simulink model "gForce_data_acquisition_ccOnline_ROS_v2_1_R2020a"  (R2022a)
settings: Solver=FixedStepAuto  StartTime=0.0  StopTime=inf  FixedStep=0.001  RelTol=1e-3
values from neighbouring files (symbols this model uses):
  k_ext = sum(u_ext)/diff_range_2    [fnc_to_be_implemented.m]
  k_flex = sum(u_flex)/diff_range_2    [fnc_to_be_implemented.m]
  M_pinv = pinv(M)    [fnc_to_be_implemented.m]
undefined symbols (not defined in the file or in its folder): gForceBLE, magnitude, W, X, Y, Z
libraries: dspfdesign x16, dspstat3 x8, robotlib x4
settings Model: SimulationMode=accelerator  Creator=Armando  LastModifiedBy=Armando
settings SolverCC: AlgebraicLoopSolver=TrustRegion
settings OptimizationCC: EnhancedBackFolding=on  PassReuseOutputArgsThreshold=0  MaxStackSize=64  OptimizeBlockOrder=speed  DifferentSizesBufferReuse=on  OptimizationCustomize=off
settings DebuggingCC: ParameterTunabilityLossMsg=error  UnconnectedInputMsg=warning  UnconnectedOutputMsg=warning  UnconnectedLineMsg=warning  SFMachineParentedDataDiag=warning
settings HardwareCC: ProdBitPerPointer=32  ProdBitPerSizeT=32  ProdBitPerPtrDiffT=32  ProdLargestAtomicFloat=None  ProdIntDivRoundTo=Undefined  ProdEndianess=Unspecified  ProdWordSize=32  ProdHWDeviceType=Generic->Unspecified (assume 32-bit Generic)  UseEmbeddedCoderFeatures=off
settings SFSimCC: MATLABDynamicMemAlloc=off  SimTargetLang=C++
settings RTWCC: SystemTargetFile=ert.tlc  HardwareBoard=Robot Operating System (ROS)  TLCOptions="-aInlineSetEventsForThisBaseRateFcn=TLC_FALSE -aSuppressMultiTaskScheduler=TLC_FALSE  -aRateBasedStepFcn=0"  TemplateMakefile=ert_default_tmf  Toolchain=Catkin  TargetLang=C++
settings CodeAppCC: ForceParamTrailComments=on  OperatorAnnotations=on
settings ERTTargetCC: ERTCustomFileBanners=off  SupportContinuousTime=on  SupportNonInlinedSFcns=on  RemoveResetFunc=off  ModelStepFunctionPrototypeControlCompliant=off

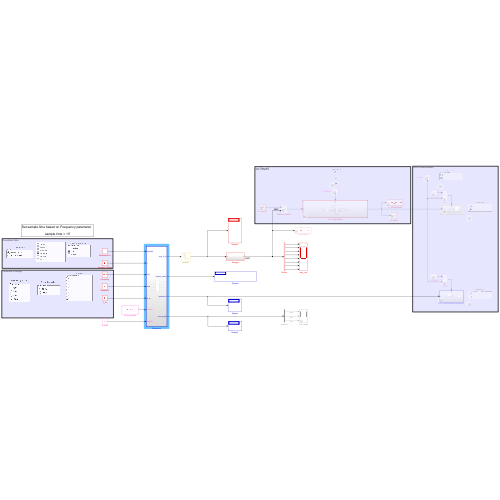
[thumbnail: Simulink's stored preview of the top-level diagram]
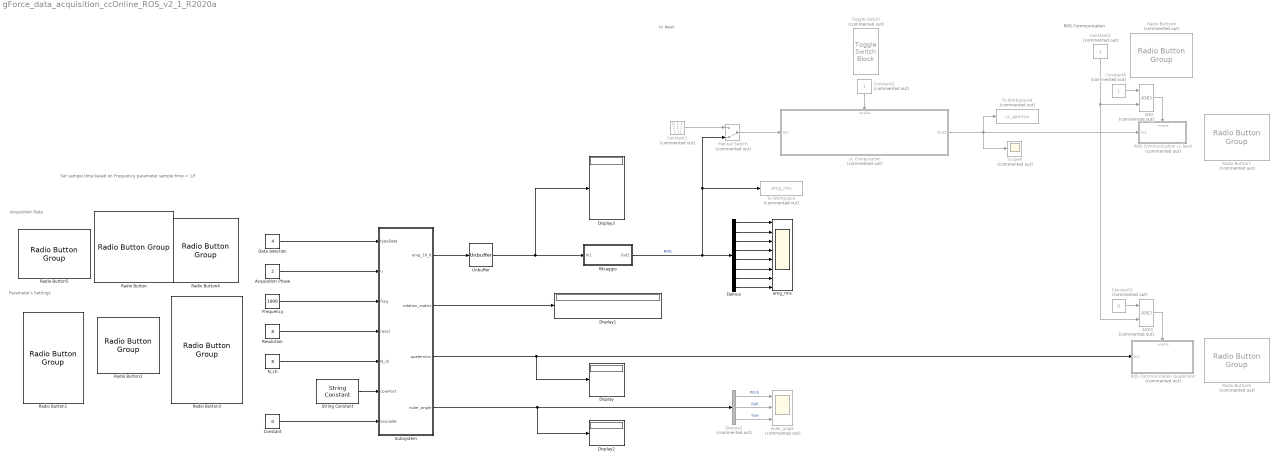
== system gForce_data_acquisition_ccOnline_ROS_v2_1_R2020a ==
  note: cc level
  note: Acquisition Data
  note: Parameter's Settings
  note: Set sample time based on Frequency parameter
      |
      | sample time = 1/f
  note: ROS Communication
  AND : Logic  Commented=on  IconShape=distinctive  AllPortsSameDT=off  OutDataTypeStr=boolean
  AND1 : Logic  Commented=on  IconShape=distinctive  AllPortsSameDT=off  OutDataTypeStr=boolean
  Acquisition Phase : Constant  Value=2  SampleTime=0.001
  Constant : Constant  Value=0
  Constant1 : Constant  Commented=on  Value=[1 1 1 1 1 1 1 1]  SampleTime=0.001
  Constant2 : Constant  Commented=on
  Constant3 : Constant  Commented=on
  Constant4 : Constant  Commented=on
  Constant5 : Constant  Commented=on  Value=0
  Data selection : Constant  Value=4  SampleTime=0.001
  Demux : Demux  Outputs=8
  Demux2 : Demux  Commented=on  Outputs=3
  Display{,1..3} (4 alike) : Display
  Frequency : Constant  Value=1000  SampleTime=0.001
  Manual Switch : ManualSwitch  Commented=on  CurrentSetting=0
  N_ch : Constant  Value=8  SampleTime=0.001
  ROS Communication cc level : Subsystem  Commented=on  TreatAsAtomicUnit=on
  ROS Communication quaternion : Subsystem  Commented=on
  Radio Button : RadioButtonGroup  SelectedLabel=EMG Raw Data  ButtonGroupName=Data Selection
      settings: Values={{'Euler Angle', 'Quaternion', 'Rotation Matrix', 'EMG Raw Data', 'EMG + Euler', 'EMG + Quat'}, [1 2 3 4 5 6]}
  Radio Button1 : RadioButtonGroup  SelectedLabel=1000  ButtonGroupName=Frequency
      settings: Values={{'100', '500', '650', '1000'}, [100 500 650 1000]}
  Radio Button2 : RadioButtonGroup  SelectedLabel=8 byte  ButtonGroupName=Resolution
      settings: Values={{'8 byte', '12 byte'}, [8 12]}
  Radio Button3 : RadioButtonGroup  SelectedLabel=8  ButtonGroupName=Numer of channels to read
      settings: Values={{'1', '2', '3', '4', '5', '6', '7', '8'}, [1 2 3 4 5 6 7 8]}
  Radio Button4 : RadioButtonGroup  SelectedLabel=Stop  ButtonGroupName=Acquisition Phase
      settings: Values={{'Acquisition', 'Stop', 'cc-level'}, [1 2 3]}
  Radio Button5 : RadioButtonGroup  SelectedLabel=gForceBLE(5CB7)  ButtonGroupName=Bracialet
      settings: Values={{'gForceBLE(5CB7)', 'gForcePro+(3BB9)'}, [0 1]}
  Radio Button6 : RadioButtonGroup  Commented=on  SelectedLabel=ON  ButtonGroupName=ROS Communication
      settings: Values={{'OFF', 'ON'}, [0 1]}
  Radio Button7 : RadioButtonGroup  Commented=on  SelectedLabel=ON  ButtonGroupName=ROS Communication cc value
      settings: Values={{'OFF', 'ON'}, [0 1]}
  Radio Button8 : RadioButtonGroup  Commented=on  SelectedLabel=OFF  ButtonGroupName=ROS Communication quaternion
      settings: Values={{'OFF', 'ON'}, [0 1]}
  Resolution : Constant  Value=8  SampleTime=0.001
  Scope6 : Scope  Commented=on
  String Constant : StringConstant  String="\"COM3\""
  Subsystem : Subsystem  TreatAsAtomicUnit=on  SystemSampleTime=0.016
  To Workspace : ToWorkspace  Commented=on  VariableName=emg_rms  SaveFormat=Timeseries  SampleTime=-1
  To Workspace4 : ToWorkspace  Commented=on  VariableName=cc_gamma  SaveFormat=Timeseries  SampleTime=-1
  Toggle Switch : ToggleSwitchBlock  Commented=on
      settings: Values={{'Off', 'On'}, [0 1]}
  Unbuffer : Unbuffer
  cc Computation : Subsystem  Commented=on
  emg_rms : Scope  NumInputPorts=8
  euler_angle : Scope  Commented=on  NumInputPorts=3
  filtraggio : Subsystem
  wires:
  Demux/8 -> emg_rms/8
  Demux2/1 -> euler_angle/1  "Pitch"
  Demux2/2 -> euler_angle/2  "Roll"
  Demux2/3 -> euler_angle/3  "Yaw"
  Subsystem/1(emg_16_8) -> Unbuffer/1
  Data selection/1 -> Subsystem/1(typeData)
  Acquisition Phase/1 -> Subsystem/2(u)
  Frequency/1 -> Subsystem/3(freq)
  Resolution/1 -> Subsystem/4(resol)
  N_ch/1 -> Subsystem/5(N_ch)
  Unbuffer/1 -> Display3/1, filtraggio/1(In1)
  Demux/1 -> emg_rms/1
  Demux/2 -> emg_rms/2
  Demux/3 -> emg_rms/3
  Demux/4 -> emg_rms/4
  Demux/5 -> emg_rms/5
  Demux/6 -> emg_rms/6
  Demux/7 -> emg_rms/7
  Subsystem/2(rotation_matrix) -> Display1/1
  String Constant/1 -> Subsystem/6(comPort)
  Constant/1 -> Subsystem/7(bracialet)
  Constant1/1 -> Manual Switch/1
  filtraggio/1(Out1) -> Manual Switch/2, To Workspace/1, Demux/1  "RMS"
  Manual Switch/1 -> cc Computation/1(In1)
  Constant2/1 -> cc Computation/Enable
  cc Computation/1(Out1) -> Scope6/1, ROS Communication cc level/1(In1), To Workspace4/1
  Subsystem/3(quaternion) -> ROS Communication quaternion/1(In1), Display/1
  AND/1 -> ROS Communication cc level/Enable
  AND1/1 -> ROS Communication quaternion/Enable
  Constant4/1 -> AND/1
  Constant5/1 -> AND1/1
  Constant3/1 -> AND1/2, AND/2
  Subsystem/4(euler_angle) -> Display2/1, Demux2/1

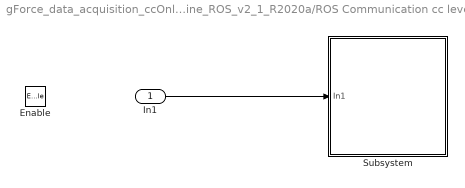
== system gForce_data_acquisition_ccOnline_ROS_v2_1_R2020a/ROS Communication cc level ==
  In1 : Inport
  Enable : EnablePort
  Subsystem : Subsystem  TreatAsAtomicUnit=on  SystemSampleTime=0.01
  wires:
  In1/1 -> Subsystem/1(In1)

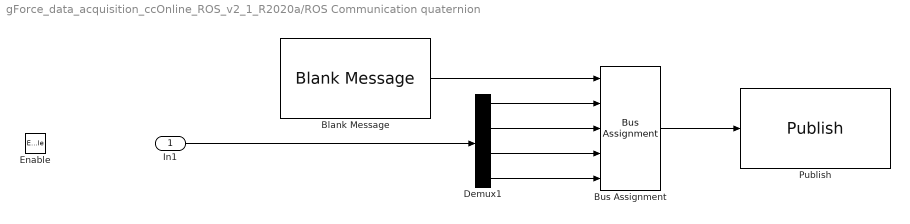
== system gForce_data_acquisition_ccOnline_ROS_v2_1_R2020a/ROS Communication quaternion ==
  In1 : Inport
  Enable : EnablePort
  Blank Message : robotlib/Blank Message  messageClass=Message  entityType=geometry_msgs/Quaternion  messageType=geometry_msgs/Quaternion  SampleTime=inf  legacyBusStruct=off
  Bus Assignment : BusAssignment  AssignedSignals=W,X,Y,Z
  Demux1 : Demux
  Publish : robotlib/Publish  topicSource=Specify your own  topic=/gForce_quaternion  messageType=geometry_msgs/Quaternion  legacyBusStruct=off  messageQueueLength=1
  wires:
  Bus Assignment/1 -> Publish/1
  Blank Message/1 -> Bus Assignment/1
  Demux1/4 -> Bus Assignment/5
  Demux1/1 -> Bus Assignment/2
  Demux1/2 -> Bus Assignment/3
  Demux1/3 -> Bus Assignment/4
  In1/1 -> Demux1/1

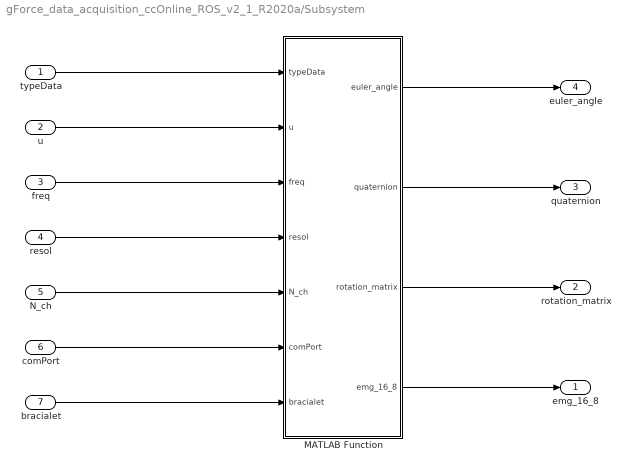
== system gForce_data_acquisition_ccOnline_ROS_v2_1_R2020a/Subsystem ==
  typeData : Inport
  u : Inport  Port=2
  freq : Inport  Port=3
  resol : Inport  Port=4
  N_ch : Inport  Port=5
  comPort : Inport  Port=6
  bracialet : Inport  Port=7
  MATLAB Function : MATLAB Function  TreatAsAtomicUnit=on  SystemSampleTime=0.016
  emg_16_8 : Outport
  rotation_matrix : Outport  Port=2
  quaternion : Outport  Port=3
  euler_angle : Outport  Port=4
  wires:
  N_ch/1 -> MATLAB Function/5(N_ch)
  freq/1 -> MATLAB Function/3(freq)
  resol/1 -> MATLAB Function/4(resol)
  u/1 -> MATLAB Function/2(u)
  MATLAB Function/4(emg_16_8) -> emg_16_8/1
  typeData/1 -> MATLAB Function/1(typeData)
  MATLAB Function/3(rotation_matrix) -> rotation_matrix/1
  MATLAB Function/2(quaternion) -> quaternion/1
  MATLAB Function/1(euler_angle) -> euler_angle/1
  comPort/1 -> MATLAB Function/6(comPort)
  bracialet/1 -> MATLAB Function/7(bracialet)

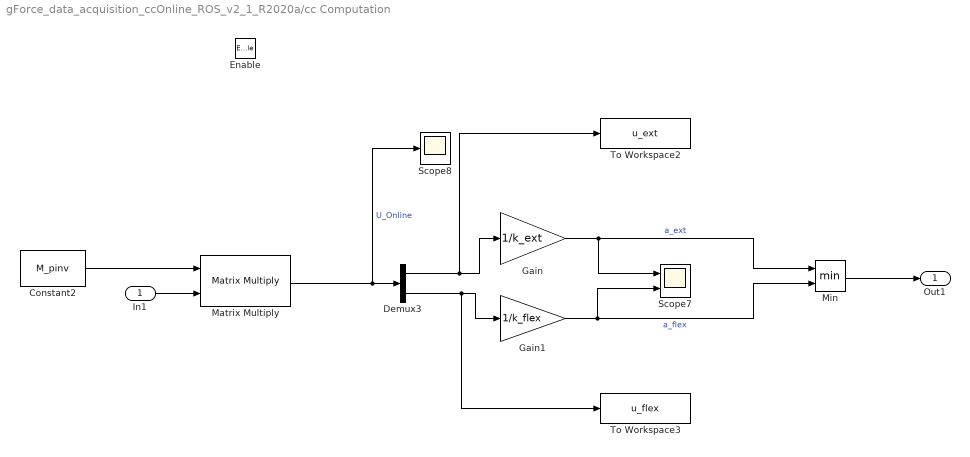
== system gForce_data_acquisition_ccOnline_ROS_v2_1_R2020a/cc Computation ==
  In1 : Inport
  Enable : EnablePort
  Constant2 : Constant  Value=M_pinv  SampleTime=0.001
  Demux3 : Demux  Outputs=2
  Gain : Gain  Gain=1/k_ext
  Gain1 : Gain  Gain=1/k_flex
  Matrix Multiply : Product  Multiplication=Matrix(*)
  Min : MinMax  Inputs=2
  Scope7 : Scope  NumInputPorts=2
  Scope8 : Scope
  To Workspace2 : ToWorkspace  VariableName=u_ext  SaveFormat=Timeseries  SampleTime=-1
  To Workspace3 : ToWorkspace  VariableName=u_flex  SaveFormat=Timeseries  SampleTime=-1
  Out1 : Outport
  wires:
  Gain1/1 -> Scope7/2, Min/2  "a_flex"
  Matrix Multiply/1 -> Demux3/1, Scope8/1  "U_Online"
  Constant2/1 -> Matrix Multiply/1
  Gain/1 -> Scope7/1, Min/1  "a_ext"
  Demux3/1 -> To Workspace2/1, Gain/1
  Min/1 -> Out1/1
  Demux3/2 -> To Workspace3/1, Gain1/1
  In1/1 -> Matrix Multiply/2

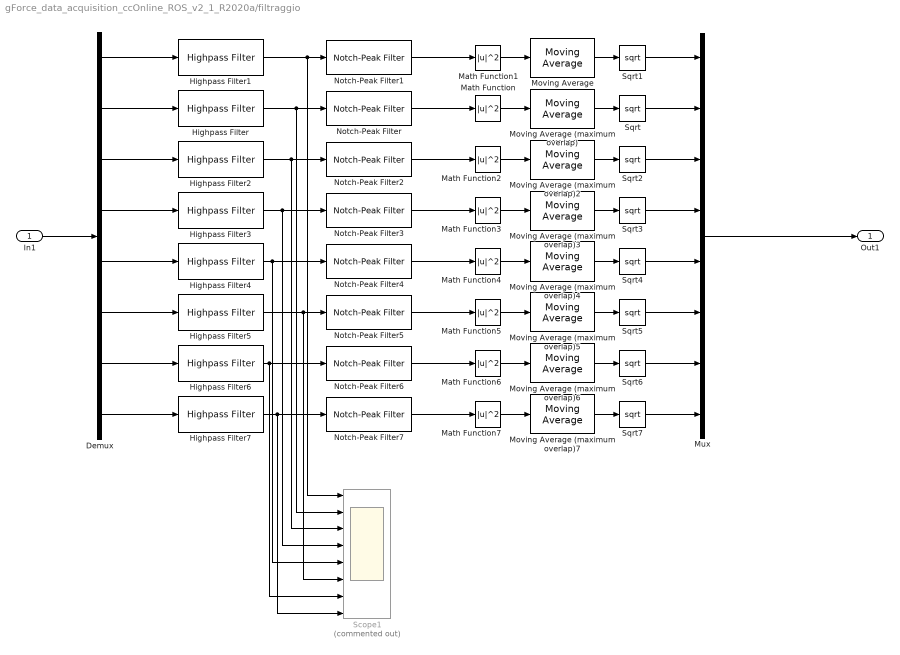
== system gForce_data_acquisition_ccOnline_ROS_v2_1_R2020a/filtraggio ==
  In1 : Inport
  Demux : Demux  Outputs=8
  Highpass Filter{,1..7} (8 alike) : dspfdesign/Highpass Filter  FilterType=FIR  DesignForMinimumOrder=on  FilterOrder=50  StopbandFrequency=15  PassbandFrequency=20  StopbandAttenuation=80  PassbandRipple=0.1  InheritSampleRate=off  SampleRate=1000  SimulateUsing=Interpreted execution  roundingMode=Floor  coeffsDataTypeStr=fixdt(1,16)
  Math Function{,1..7} (8 alike) : Math  Operator=magnitude^2  SignedPower=on
  Moving Average (maximum overlap){,2..7} (7 alike) : dspstat3/Moving Average  Method=Sliding window  ForgettingFactorPort=off  SpecifyWindowLength=on  WindowLength=200  ForgettingFactor=0.9  SimulateUsing=Code generation
  Moving Average : dspstat3/Moving Average  Method=Sliding window  ForgettingFactorPort=off  SpecifyWindowLength=on  WindowLength=200  ForgettingFactor=0.9  SimulateUsing=Code generation
  Mux : Mux  Inputs=8
  Notch-Peak Filter{,1..7} (8 alike) : dspfdesign/Notch-Peak Filter  Specification=Quality factor and center frequency  BandwidthPort=off  Bandwidth=2205  QualityFactorPort=off  QualityFactor=5  CenterFrequencyPort=off  CenterFrequency=50  BandwidthCoefficientPort=off  BandwidthCoefficient=0.72654  CenterFrequencyCoefficientPort=off  CenterFrequencyCoefficient=0  Output=Notch  InheritSampleRate=off  SampleRate=1000  SimulateUsing=Code generation
      settings: SourceProductBaseCode=DS
  Scope1 : Scope  Commented=on  NumInputPorts=8
  Sqrt{,1..7} (8 alike) : Sqrt
  Out1 : Outport
  wires:
  In1/1 -> Demux/1
  Highpass Filter/1 -> Scope1/2, Notch-Peak Filter/1
  Notch-Peak Filter/1 -> Math Function/1
  Math Function/1 -> Moving Average (maximum overlap)/1
  Moving Average (maximum overlap)/1 -> Sqrt/1
  Mux/1 -> Out1/1
  Moving Average/1 -> Sqrt1/1
  Math Function1/1 -> Moving Average/1
  Notch-Peak Filter1/1 -> Math Function1/1
  Highpass Filter1/1 -> Scope1/1, Notch-Peak Filter1/1
  Moving Average (maximum overlap)2/1 -> Sqrt2/1
  Math Function2/1 -> Moving Average (maximum overlap)2/1
  Notch-Peak Filter2/1 -> Math Function2/1
  Highpass Filter2/1 -> Scope1/3, Notch-Peak Filter2/1
  Moving Average (maximum overlap)3/1 -> Sqrt3/1
  Math Function3/1 -> Moving Average (maximum overlap)3/1
  Notch-Peak Filter3/1 -> Math Function3/1
  Highpass Filter3/1 -> Scope1/4, Notch-Peak Filter3/1
  Moving Average (maximum overlap)4/1 -> Sqrt4/1
  Math Function4/1 -> Moving Average (maximum overlap)4/1
  Notch-Peak Filter4/1 -> Math Function4/1
  Highpass Filter4/1 -> Scope1/5, Notch-Peak Filter4/1
  Moving Average (maximum overlap)5/1 -> Sqrt5/1
  Math Function5/1 -> Moving Average (maximum overlap)5/1
  Notch-Peak Filter5/1 -> Math Function5/1
  Highpass Filter5/1 -> Scope1/6, Notch-Peak Filter5/1
  Moving Average (maximum overlap)6/1 -> Sqrt6/1
  Math Function6/1 -> Moving Average (maximum overlap)6/1
  Notch-Peak Filter6/1 -> Math Function6/1
  Highpass Filter6/1 -> Scope1/7, Notch-Peak Filter6/1
  Moving Average (maximum overlap)7/1 -> Sqrt7/1
  Math Function7/1 -> Moving Average (maximum overlap)7/1
  Notch-Peak Filter7/1 -> Math Function7/1
  Highpass Filter7/1 -> Scope1/8, Notch-Peak Filter7/1
  Demux/1 -> Highpass Filter1/1
  Demux/2 -> Highpass Filter/1
  Demux/3 -> Highpass Filter2/1
  Demux/4 -> Highpass Filter3/1
  Demux/5 -> Highpass Filter4/1
  Demux/6 -> Highpass Filter5/1
  Demux/7 -> Highpass Filter6/1
  Demux/8 -> Highpass Filter7/1
  Sqrt/1 -> Mux/2
  Sqrt2/1 -> Mux/3
  Sqrt3/1 -> Mux/4
  Sqrt4/1 -> Mux/5
  Sqrt5/1 -> Mux/6
  Sqrt6/1 -> Mux/7
  Sqrt7/1 -> Mux/8
  Sqrt1/1 -> Mux/1

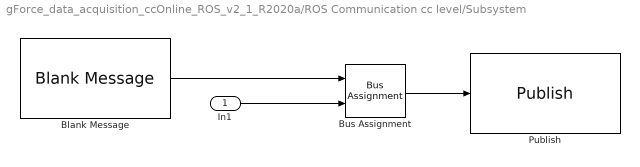
== system gForce_data_acquisition_ccOnline_ROS_v2_1_R2020a/ROS Communication cc level/Subsystem ==
  In1 : Inport
  Blank Message : robotlib/Blank Message  messageClass=Message  entityType=std_msgs/Float64  messageType=std_msgs/Float64  SampleTime=inf  legacyBusStruct=off
  Bus Assignment : BusAssignment  AssignedSignals=Data
  Publish : robotlib/Publish  topicSource=Specify your own  topic=/gForce_cc  messageType=std_msgs/Float64  legacyBusStruct=off  messageQueueLength=1
  wires:
  Blank Message/1 -> Bus Assignment/1
  In1/1 -> Bus Assignment/2
  Bus Assignment/1 -> Publish/1

== matlab function gForce_data_acquisition_ccOnline_ROS_v2_1_R2020a/Subsystem/MATLAB Function ==
  data: euler_angle output; quaternion output; rotation_matrix output; typeData input; emg_16_8 output; u input; freq input; resol input; N_ch input; comPort input; bracialet input
%%%%%%%%%
%
%   Questa funzione funge da filtraggio del pacchetto di dati inviato
%   dal braccialetto
%
%%%%%%%%%
%%%%%%%%%%%%%%%%%%%%%%%%%%%
%   This function acts as data pack filter sent from the bracialet
%   Input:
%       1 - [scalar]	Data selection [1,2,3,4,5,6]        
%		2 - [scalar]	Acquisition's Phase [1,2,3] 
%		3 - [scalar]	Acquisition's frequency [100,500,650,1000]
%		4 - [scalar]	Acquisition's resolution [8bits , 12bits] 
%		5 - [scalar]	Acquisition's channels [1,2,3,4,5,6,7,8]  
%	Output:
%       1 - [row vector 1x3]   first byte of data pack w/o header
%		2 - [row vector 1x4]   first byte of data pack w/o header
%       3 - [row vector 1x9]   first byte of data pack w/o header 
%		4 - [matrix 16x8]   data pack w/o header organized in matrix form
%       
%   For any further information please read the <information_file> or contact
%       - Armando Amerì to armando.ameri@studio.unibo.it
%       - Roberto Meattini to roberto.meattini2@unibo.it
%%%%%%%%%%%%%%%%%%%%%%%%%%%

function [euler_angle,quaternion,rotation_matrix,emg_16_8] = fcn(typeData,u,freq,resol,N_ch,comPort,bracialet)

%--- Inizializzation
% data1 = zeros(3,1);   %euler angle
% data2 = zeros(4,1);     %quaternion
% data3 = zeros(9,1);     %rotation
data4 = zeros(141,1);   %emg

% data_8_in_row = zeros(1,8);
euler_angle = zeros(1,3);
quaternion = zeros(1,4);
rotation_matrix = zeros(1,9);
emg_16_8 = zeros(16,8);

    if typeData == 1
        %disp('Euler Angle:')
        euler_angle = Data_Pack_euler_angle(u,comPort,bracialet)'
    elseif typeData == 2
        %disp('Quaternion:')
        quaternion = Data_Pack_quaternion(u,comPort,bracialet)'
    elseif typeData == 3
        %disp('Rotation matrix:')
        rotation_matrix = Data_Pack_rotation_matrix(u,comPort,bracialet)'
    elseif typeData == 4
        j = 1;
        %EMG_Raw_Data_Pack
        data4 = Data_Pack_EMG_Raw(u,freq,resol,N_ch,comPort,bracialet);
        %EMG_Raw_Data_First_8
        %data_8_in_row = data0(14:21,1)';
        %EMG_Raw_Data_Pack_16
        for i = 14:8:141
            emg_16_8(j,:) = data4(i:i+7,1)';
            j = j +1;
        end
    elseif typeData == 5
        disp('EMG + Euler Angle to be programmed')
    elseif typeData == 6
        disp('EMG + Quaternion to be programmed')  
    else
        disp('to be programmed')
    end
end
